simulink model "circuito_RLC_apostila_kraus_exemplo5"  (R2023b)
settings: Solver=VariableStepAuto  StartTime=0.0  StopTime=3.0  RelTol=1e-3
settings Model: Creator=thiag  LastModifiedBy=thiag

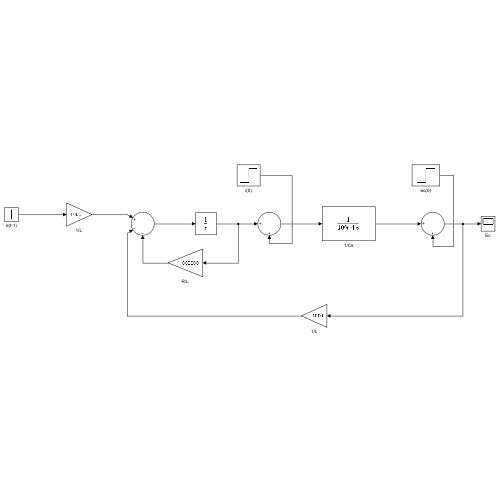
[thumbnail: Simulink's stored preview of the top-level diagram]
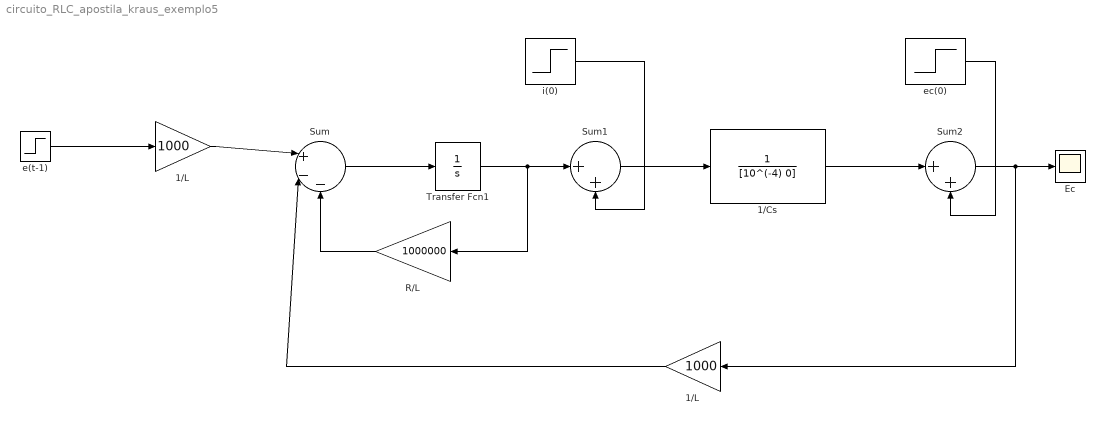
== system circuito_RLC_apostila_kraus_exemplo5 ==
  1/Cs : TransferFcn  Denominator=[10^(-4) 0]
  1/L : Gain  Gain=1000
  "1/L " : Gain  Gain=1000
  Ec : Scope
  R/L : Gain  Gain=1000000
  Sum : Sum  Inputs=|+--
  Sum1 : Sum  Inputs=|++
  Sum2 : Sum  Inputs=|++
  Transfer Fcn1 : TransferFcn  Denominator=[1 0]
  e(t-1) : Step  SampleTime=0
  ec(0) : Step  Time=0  After=0.5  SampleTime=0
  i(0) : Step  Time=0  After=0.001  SampleTime=0
  wires:
  e(t-1)/1 -> "1/L "/1
  "1/L "/1 -> Sum/1
  Sum2/1 -> 1/L/1, Ec/1
  1/L/1 -> Sum/2
  R/L/1 -> Sum/3
  Transfer Fcn1/1 -> R/L/1, Sum1/1
  Sum/1 -> Transfer Fcn1/1
  Sum1/1 -> 1/Cs/1
  1/Cs/1 -> Sum2/1
  i(0)/1 -> Sum1/2
  ec(0)/1 -> Sum2/2
